simulink model "s2dot2_75ziqinglinjifenqi"  (R2023b)
settings: Solver=VariableStepAuto  StartTime=0.0  StopTime=30  RelTol=1e-3
settings Model: Creator=lxj  LastModifiedBy=lxj

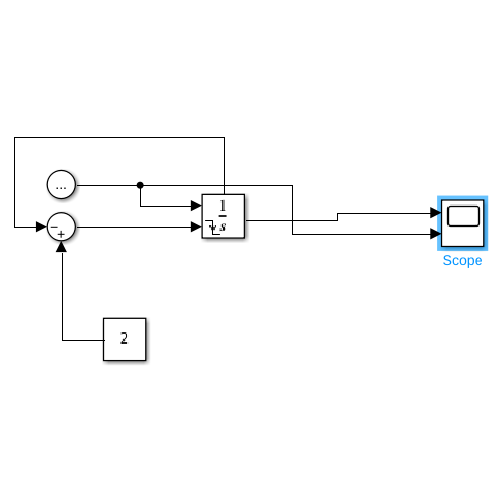
[thumbnail: Simulink's stored preview of the top-level diagram]
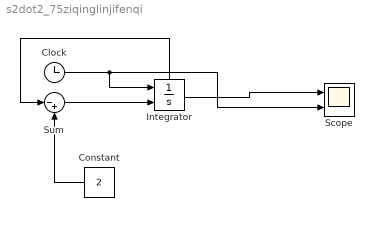
== system s2dot2_75ziqinglinjifenqi ==
  Clock : Clock
  Constant : Constant  Value=2
  Integrator : Integrator  ExternalReset=falling  ShowStatePort=on
  Scope : Scope  NumInputPorts=2
  Sum : Sum  Inputs=|-+
  wires:
  Integrator/1 -> Scope/1
  Clock/1 -> Scope/2, Integrator/1
  Sum/1 -> Integrator/2
  Constant/1 -> Sum/2
  Integrator/State -> Sum/1
